simulink model "Hierarchy4"  (Simulink 8.7)
settings: Solver=ode45  StartTime=0.0  StopTime=10.0  RelTol=1e-3
settings Model: Creator=scaife  LastModifiedBy=bourbouh  ExtModeAutoUpdateStatusClock=off
settings DataIOCC: SignalLoggingSaveFormat=ModelDataLogs  SignalLoggingName=sigsOut
settings DebuggingCC: SaveWithParameterizedLinksMsg=none  SignalResolutionControl=TryResolveAllWithWarning  MultiTaskDSMMsg=warning  MultiTaskCondExecSysMsg=none
settings HardwareCC: TargetUnknown=on
settings SFSimCC: SimParseCustomCode=off
settings GRTTargetCC: GeneratePreprocessorConditionals=Use local settings  CombineOutputUpdateFcns=off  GRTInterface=on

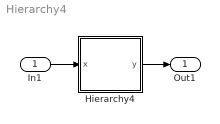
== system Hierarchy4 ==
  In1 : Inport
  Hierarchy4 : Stateflow chart  TreatAsAtomicUnit=on
  Out1 : Outport
  wires:
  In1/1 -> Hierarchy4/1(x)
  Hierarchy4/1(y) -> Out1/1

== stateflow chart Hierarchy4 ==
  state A/
    en: y=1;
  state B/
    en: y=2;
  (default) -> A [order 1] : [x==0]
  (default) -> B [order 2] : [x<>0]
  data: x input int32; y output int32
